simulink model "external_memory_test"  (R2020b)
settings: Solver=FixedStepDiscrete  StartTime=0.0  StopTime=80  RelTol=1e-3
InitFcn:
  | Feature_Width = 64;
  | Feature_Height = 64;
  | Weight_Width = 3;
  | Weight_Height = 3;
  | external_memory_test_init;
values from neighbouring files (symbols this model uses):
  Burst_Length = Feature_Weight_Length    [external_memory_test_init.m]
  byPass = 1    [external_memory_test_init.m]
  Conv_Padding = 0    [external_memory_test_init.m]
  Conv_Stride = 1    [external_memory_test_init.m]
  DDR_Depth = Weight_Length + Feature_Length + outFeature_Length    [external_memory_test_init.m]
  ddrInitData = single((rand(1,DDR_Depth)))    [external_memory_test_init.m]
  Duty_Cycle = 0.5    [external_memory_test_init.m]
  Feature_Area = Feature_Width * Feature_Height    [external_memory_test_init.m]
  Feature_Length = Phase_In * Feature_Area    [external_memory_test_init.m]
  inChannel = 3    [external_memory_test_init.m]
  outChannel = 2    [external_memory_test_init.m]
  outFeature_Length = outFeature_Width * outFeature_Height * Phase_Out    [external_memory_test_init.m]
  Pool_Stride = 2    [external_memory_test_init.m]
  Pool_Width = 2    [external_memory_test_init.m]
  Tc = 1    [external_memory_test_init.m]
  Ti = 1    [external_memory_test_init.m]
  To = 1    [external_memory_test_init.m]
  Tr = 1    [external_memory_test_init.m]
  Weight_Length = Phase_In * Weight_Area * Phase_Out    [external_memory_test_init.m]
undefined symbols (not defined in the file or in its folder): Conv_Step, Pool_Step, sigbuilder_block
libraries: hdlsllib x85, simulink x44, visionhdlutilities x16
(part 1 of 6)
settings Model: DataTypeOverride=Off  Creator=Xiao  LastModifiedBy=Xiao
settings SolverCC: AutoInsertRateTranBlk=on
settings OptimizationCC: BlockReduction=off  ConditionallyExecuteInputs=off  DefaultParameterBehavior=Inlined
settings DebuggingCC: AlgebraicLoopMsg=error  SingleTaskRateTransMsg=error
settings HardwareCC: ProdBitPerPointer=32  ProdBitPerSizeT=32  ProdBitPerPtrDiffT=32  ProdLargestAtomicFloat=None  ProdIntDivRoundTo=Undefined  ProdEndianess=Unspecified  ProdWordSize=32  ProdHWDeviceType=ASIC/FPGA->ASIC/FPGA  TargetBitPerPointer=64  TargetBitPerSizeT=64  TargetBitPerPtrDiffT=64  TargetLongLongMode=on  TargetIntDivRoundTo=Zero  TargetEndianess=LittleEndian  TargetWordSize=64  TargetHWDeviceType=Custom Processor->MATLAB Host Computer  ProdEqTarget=off

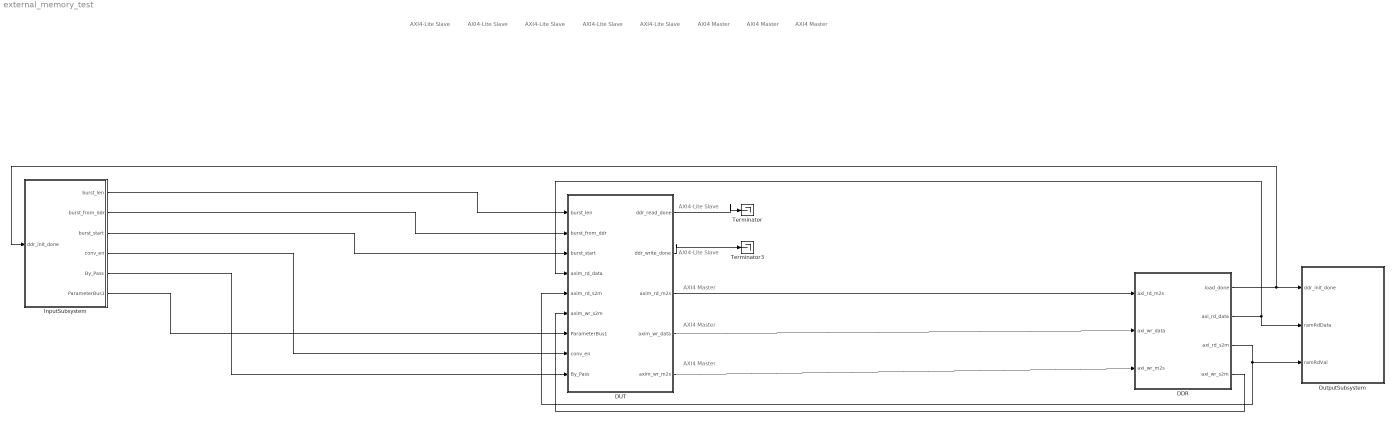
== system external_memory_test ==
  note: AXI4 Master
  note: AXI4-Lite Slave
  note: AXI4-Lite Slave
  note: AXI4-Lite Slave
  note: AXI4 Master
  note: AXI4 Master
  note: AXI4-Lite Slave
  note: AXI4-Lite Slave
  note: AXI4 Master
  note: AXI4-Lite Slave
  note: AXI4 Master
  note: AXI4 Master
  note: AXI4-Lite Slave
  DDR : Subsystem  mask{DDR3_DEPTH=DDR_Depth, INIT_DDR3=on, INIT_ADDR=0, INIT_DATA=ddrInitData(1:DDR_Depth), OutDataTypeStr=uint32, READY_DUTY_CYL=Duty_Cycle, toggle=off}
      mask prompts: DDR3_DEPTH "DDR3 DEPTH"; INIT_DDR3 "Initialize DDR3"; INIT_ADDR "DDR3 Initial Address"; INIT_DATA "DDR3 Initialization data"; OutDataTypeStr "Simulink:blkprm_prompts:UNIFIEDDATATYPE"; READY_DUTY_CYL "READY Duty Cycle"; toggle "Read Valid Toggling"
      mask help: DDR3 Simulation model
      mask init:
      | if(DDR3_DEPTH<=1)
      |     error('DDR size should be greater than 1' )  
      | end
      | 
      | if(READY_DUTY_CYL>1)
      |   error('should be less than 1' )  
      | end
      |    
      | 
      | %%Initialization Value
      | if(INIT_DDR3==true)
      |     if(isempty(INIT_ADDR))
      |      error('Enter Initial address' )  
      |     end   
      | end
      mask Callback INIT_DDR3:
      | % Get the mask parameter values. This is a cell
      | %   array of character vectors.
      | maskStr = get_param(gcb,'INIT_DDR3');
      | 
      | % The pop-up menu is the first mask parameter.
      | %   Check the value selected in the pop-up
      | if strcmp(maskStr,'on')
      | 
      |     % Set the visibility of both parameters on when
      |     %   User-defined is selected in the pop-up.
      | 
      |     set_param(gcb,'MaskEnables',{'on','on','on','on','on','on','on'});
      | 
      | else
      | 
      |     % Turn off the visibility of the Value field
      |     %   when User-defined is not selected.
      | 
      |     set_param(gcb,'MaskEnables',{'on','on','off','off','on','on','on'});
      | 
      |     % Set the character vector in the Values field equal to the
      |     % character vector selected in the Gain pop-up menu.
      | 
      |     %maskStr{2}=maskStr{1};
      | 
      | end
      mask TypeOptions OutDataTypeStr: axi_wr_data/OutDataTypeStr | axi_rd_data/OutDataTypeStr
      mask DialogControl DescGroupVar Prompt: DDR
      mask DialogControl DDR3_INIT Prompt: DDR3 Initialization
      mask DialogControl PARAM_GROUP Prompt: DDR3 Initialization Parameters
      mask DialogControl OutDataTypeStr Prompt: Data type:
      mask DialogControl READY_DUTY_CYL Tooltip: between 0 to 1
  DUT : Subsystem  TreatAsAtomicUnit=on
  InputSubsystem : Subsystem
  OutputSubsystem : Subsystem
  Terminator : Terminator
  Terminator3 : Terminator
  wires:
  DDR/2(axi_rd_data) -> OutputSubsystem/2(ramRdData), DUT/4(axim_rd_data)
  DDR/4(axi_wr_s2m) -> DUT/6(axim_wr_s2m)
  DUT/4(axim_wr_data) -> DDR/2(axi_wr_data)
  DUT/5(axim_wr_m2s) -> DDR/3(axi_wr_m2s)
  DDR/3(axi_rd_s2m) -> OutputSubsystem/3(ramRdVal), DUT/5(axim_rd_s2m)
  DUT/1(ddr_read_done) -> Terminator/1
  DUT/2(ddr_write_done) -> Terminator3/1
  DUT/3(axim_rd_m2s) -> DDR/1(axi_rd_m2s)
  InputSubsystem/2(burst_from_ddr) -> DUT/2(burst_from_ddr)
  InputSubsystem/3(burst_start) -> DUT/3(burst_start)
  InputSubsystem/1(burst_len) -> DUT/1(burst_len)
  DDR/1(load_done) -> OutputSubsystem/1(ddr_init_done), InputSubsystem/1(ddr_init_done)
  InputSubsystem/4(conv_en) -> DUT/8(conv_en)
  InputSubsystem/5(By_Pass) -> DUT/9(By_Pass)
  InputSubsystem/6(ParameterBus1) -> DUT/7(ParameterBus1)

== system external_memory_test/DDR ==
  axi_rd_m2s : Inport
  axi_wr_data : Inport  Port=2  OutDataTypeStr=uint32
  axi_wr_m2s : Inport  Port=3
  Bit Slice1 : hdlsllib/Logic and Bit Operations/Bit Slice  lidx=15  ridx=0
  Bus Creator : BusCreator  Inputs=2
  Bus Creator1 : BusCreator  Inputs=2
  Bus Selector : BusSelector  OutputSignals=rd_addr,rd_len,rd_avalid
  Bus Selector1 : BusSelector  OutputSignals=wr_addr,wr_len,wr_valid
  Constant : Constant  OutDataTypeStr=boolean  SampleTime=-1
  Delay : Delay
  Delay1 : Delay  DelayLength=1
  Delay2 : Delay  DelayLength=1
  Delay3 : Delay  DelayLength=1
  MATLAB System : MATLABSystem  System=hdl.RAM  RAMType=Simple dual port  WriteOutputValue=New data  RAMInitialValue=0  SimulateUsing=Code generation
      mask Type: hdl.RAM
      mask Display:
      | disp(['Simple' char(10) 'Dual Port' char(10) 'RAM']);
      | port_label('input',1,'din');
      | port_label('input',2,'wr_addr');
      | port_label('input',3,'wr_en');
      | port_label('input',4,'rd_addr');
      | port_label('output',1,'rd_dout');
  ddr_ready : Subsystem
  load_init_data : MATLAB Function  TreatAsAtomicUnit=on
  rdLogic : Subsystem
  wrLogic : Subsystem
  wr_addr-3 : Delay  DelayLength=1
  load_done : Outport  VectorParamsAs1DForOutWhenUnconnected=off
  axi_rd_data : Outport  Port=2  OutDataTypeStr=uint32  VectorParamsAs1DForOutWhenUnconnected=off
  axi_rd_s2m : Outport  Port=3  VectorParamsAs1DForOutWhenUnconnected=off
  axi_wr_s2m : Outport  Port=4  VectorParamsAs1DForOutWhenUnconnected=off
  wires:
  Bit Slice1/1 -> wr_addr-3/1
  Delay1/1 -> axi_rd_data/1
  load_init_data/4(ram_wr_enb) -> MATLAB System/3  "ddr_wr_en"
  load_init_data/3(ram_wr_add) -> Bit Slice1/1
  load_init_data/1(load_done) -> ddr_ready/Enable, load_done/1
  MATLAB System/1 -> Delay1/1  "ddr_dout"
  rdLogic/1(ram_rd_addr) -> MATLAB System/4  "ddr_rd_addr"
  wrLogic/1(ram_wr_addr) -> load_init_data/2(axi_wr_add)
  wrLogic/2(ram_wr_enb) -> load_init_data/3(axi_wr_val)
  wr_addr-3/1 -> MATLAB System/2  "ddr_wr_addr"
  Bus Selector/2 -> rdLogic/2(axim_rd_len)  "<rd_len>"
  Bus Selector/1 -> rdLogic/1(axim_rd_addr)  "<rd_addr>"
  Constant/1 -> rdLogic/4(axi_rd_dready)  "<rd_dready>"
  axi_rd_m2s/1 -> Bus Selector/1
  Bus Selector/3 -> rdLogic/3(axim_rd_avalid)  "<rd_avalid>"
  Bus Selector1/1 -> wrLogic/2(axi_addr)  "<wr_addr>"
  axi_wr_m2s/1 -> Delay3/1
  Bus Selector1/3 -> wrLogic/4(axi_wr_enb)  "<wr_valid>"
  Bus Selector1/2 -> wrLogic/3(axi_wr_len)  "<wr_len>"
  rdLogic/2(axim_rd_aready) -> Bus Creator/1  "rd_aready"
  Bus Creator/1 -> axi_rd_s2m/1
  rdLogic/3(axim_rd_dvalid) -> Bus Creator/2  "rd_dvalid"
  ddr_ready/1(rdy_out) -> Delay/1, wrLogic/1(ddr_rdy)
  Bus Creator1/1 -> axi_wr_s2m/1
  wrLogic/3(axi_wr_ack) -> Bus Creator1/2  "wr_complete"
  Delay/1 -> Bus Creator1/1  "wr_ready"
  load_init_data/2(ram_wr_data) -> MATLAB System/1  "ddr_din"
  axi_wr_data/1 -> Delay2/1
  Delay2/1 -> load_init_data/1(axi_wr_data)
  Delay3/1 -> Bus Selector1/1

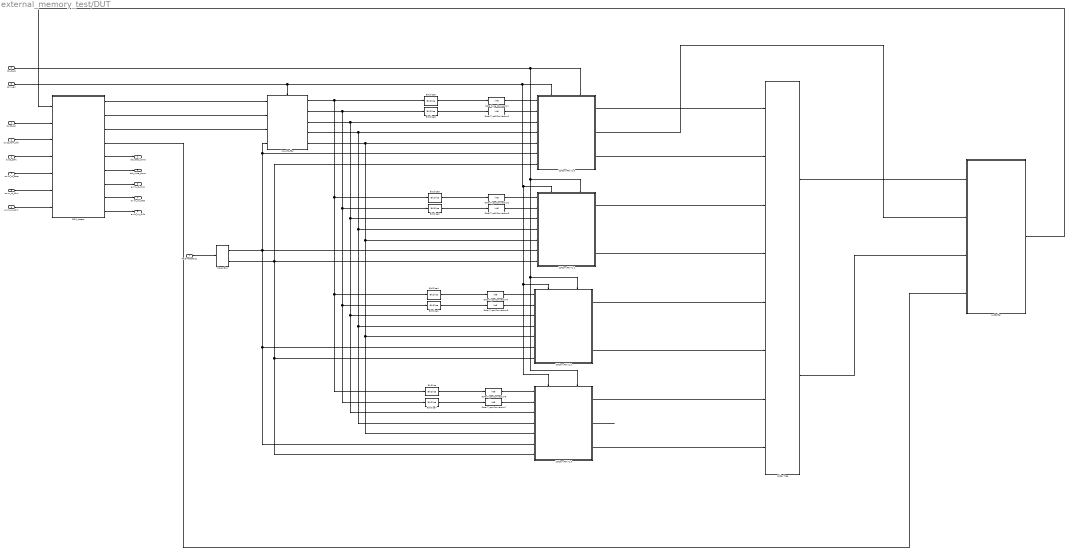
== system external_memory_test/DUT ==
  burst_len : Inport
  burst_from_ddr : Inport  Port=2
  burst_start : Inport  Port=3
  axim_rd_data : Inport  Port=4
  axim_rd_s2m : Inport  Port=5
  axim_wr_s2m : Inport  Port=6
  ParameterBus1 : Inport  Port=7
  conv_en : Inport  Port=8
  By_Pass : Inport  Port=9
  2DConvPE V1.0 : Subsystem
      settings: PortSchema="{\"entries\":[{\"content\":{\"sides\":[{\"content\":{\"connectorIds\":[\"In1\",\"In2\",\"In3\",\"In4\",\"In5\",\"In6\",\"In7\"]},\"type\":\"ConnectorPlacement.EquallySpacedRectSide\",\"uuid\":\"72a132f7-3e47-4ef1-8d79-baadbeb84817\"},{\"content\":{\"connectorIds\":[\"Out1\",\"Out2\",\"Out3\"],\"side\":\"RIGHT\"},\"type\":\"ConnectorPlacement.EquallySpacedRectSide\",\"uuid\":\"2df9bf31-2175-4d97-aafa-a0227f37f2af\"},{\"content\":{\"connectorIds\":[\"In8\",\"In9\"],\"side\":\"TOP\"},\"type\":\"ConnectorPlacement.EquallySpacedRectSide\",\"uuid\":\"1b8495b8-ab7c-42d9-b044-413e20debbac\"},{\"content\":{\"connectorIds\":[],\"side\":\"BOTTOM\"},\"type\":\"ConnectorPlacement.EquallySpacedRectSide\",\"uuid\":\"e68361ac-7f7b-4816-948a-9cecfdd8f729\"},{\"content\":{\"connectorIds\":[],\"side\":\"HIDDEN\"},\"type\":\"ConnectorPlacement.EquallySpacedRectSide\",\"uuid\":\"818be012-dd2c-438f-8537-4d3d95a16bb4\"}]},\"type\":\"ConnectorPlacement.EquallySpacedConnector\",\"uuid\":\"cbadf64c-68f0-4765-b1bf-d60756169ff2\"}],\"packageUris\":[\"http://schema.mathworks.com/mf0/Connector/R2020b\"],\"version\":\"1.0\"}"
  2DConvPE V1.1 : Subsystem
      settings: PortSchema="{\"entries\":[{\"content\":{\"sides\":[{\"content\":{\"connectorIds\":[\"In1\",\"In2\",\"In3\",\"In4\",\"In5\",\"In6\",\"In7\"]},\"type\":\"ConnectorPlacement.EquallySpacedRectSide\",\"uuid\":\"72a132f7-3e47-4ef1-8d79-baadbeb84817\"},{\"content\":{\"connectorIds\":[\"Out1\",\"Out2\",\"Out3\"],\"side\":\"RIGHT\"},\"type\":\"ConnectorPlacement.EquallySpacedRectSide\",\"uuid\":\"2df9bf31-2175-4d97-aafa-a0227f37f2af\"},{\"content\":{\"connectorIds\":[\"In8\",\"In9\"],\"side\":\"TOP\"},\"type\":\"ConnectorPlacement.EquallySpacedRectSide\",\"uuid\":\"1b8495b8-ab7c-42d9-b044-413e20debbac\"},{\"content\":{\"connectorIds\":[],\"side\":\"BOTTOM\"},\"type\":\"ConnectorPlacement.EquallySpacedRectSide\",\"uuid\":\"e68361ac-7f7b-4816-948a-9cecfdd8f729\"},{\"content\":{\"connectorIds\":[],\"side\":\"HIDDEN\"},\"type\":\"ConnectorPlacement.EquallySpacedRectSide\",\"uuid\":\"818be012-dd2c-438f-8537-4d3d95a16bb4\"}]},\"type\":\"ConnectorPlacement.EquallySpacedConnector\",\"uuid\":\"cbadf64c-68f0-4765-b1bf-d60756169ff2\"}],\"packageUris\":[\"http://schema.mathworks.com/mf0/Connector/R2020b\"],\"version\":\"1.0\"}"
  2DConvPE V1.2 : Subsystem
      settings: PortSchema="{\"entries\":[{\"content\":{\"sides\":[{\"content\":{\"connectorIds\":[\"In1\",\"In2\",\"In3\",\"In4\",\"In5\",\"In6\",\"In7\"]},\"type\":\"ConnectorPlacement.EquallySpacedRectSide\",\"uuid\":\"72a132f7-3e47-4ef1-8d79-baadbeb84817\"},{\"content\":{\"connectorIds\":[\"Out1\",\"Out2\",\"Out3\"],\"side\":\"RIGHT\"},\"type\":\"ConnectorPlacement.EquallySpacedRectSide\",\"uuid\":\"2df9bf31-2175-4d97-aafa-a0227f37f2af\"},{\"content\":{\"connectorIds\":[\"In8\",\"In9\"],\"side\":\"TOP\"},\"type\":\"ConnectorPlacement.EquallySpacedRectSide\",\"uuid\":\"1b8495b8-ab7c-42d9-b044-413e20debbac\"},{\"content\":{\"connectorIds\":[],\"side\":\"BOTTOM\"},\"type\":\"ConnectorPlacement.EquallySpacedRectSide\",\"uuid\":\"e68361ac-7f7b-4816-948a-9cecfdd8f729\"},{\"content\":{\"connectorIds\":[],\"side\":\"HIDDEN\"},\"type\":\"ConnectorPlacement.EquallySpacedRectSide\",\"uuid\":\"818be012-dd2c-438f-8537-4d3d95a16bb4\"}]},\"type\":\"ConnectorPlacement.EquallySpacedConnector\",\"uuid\":\"cbadf64c-68f0-4765-b1bf-d60756169ff2\"}],\"packageUris\":[\"http://schema.mathworks.com/mf0/Connector/R2020b\"],\"version\":\"1.0\"}"
  2DConvPE V1.3 : Subsystem
      settings: PortSchema="{\"entries\":[{\"content\":{\"sides\":[{\"content\":{\"connectorIds\":[\"In1\",\"In2\",\"In3\",\"In4\",\"In5\",\"In6\",\"In7\"]},\"type\":\"ConnectorPlacement.EquallySpacedRectSide\",\"uuid\":\"72a132f7-3e47-4ef1-8d79-baadbeb84817\"},{\"content\":{\"connectorIds\":[\"Out1\",\"Out2\",\"Out3\"],\"side\":\"RIGHT\"},\"type\":\"ConnectorPlacement.EquallySpacedRectSide\",\"uuid\":\"2df9bf31-2175-4d97-aafa-a0227f37f2af\"},{\"content\":{\"connectorIds\":[\"In8\",\"In9\"],\"side\":\"TOP\"},\"type\":\"ConnectorPlacement.EquallySpacedRectSide\",\"uuid\":\"1b8495b8-ab7c-42d9-b044-413e20debbac\"},{\"content\":{\"connectorIds\":[],\"side\":\"BOTTOM\"},\"type\":\"ConnectorPlacement.EquallySpacedRectSide\",\"uuid\":\"e68361ac-7f7b-4816-948a-9cecfdd8f729\"},{\"content\":{\"connectorIds\":[],\"side\":\"HIDDEN\"},\"type\":\"ConnectorPlacement.EquallySpacedRectSide\",\"uuid\":\"818be012-dd2c-438f-8537-4d3d95a16bb4\"}]},\"type\":\"ConnectorPlacement.EquallySpacedConnector\",\"uuid\":\"cbadf64c-68f0-4765-b1bf-d60756169ff2\"}],\"packageUris\":[\"http://schema.mathworks.com/mf0/Connector/R2020b\"],\"version\":\"1.0\"}"
  Adder Tree : Subsystem
  Bit Slice : hdlsllib/Logic and Bit Operations/Bit Slice  lidx=7  ridx=0
      settings: SourceProductBaseCode=SL
  Bit Slice1 : hdlsllib/Logic and Bit Operations/Bit Slice  lidx=15  ridx=8
      settings: SourceProductBaseCode=SL
  Bit Slice2 : hdlsllib/Logic and Bit Operations/Bit Slice  lidx=23  ridx=16
      settings: SourceProductBaseCode=SL
  Bit Slice3 : hdlsllib/Logic and Bit Operations/Bit Slice  lidx=31  ridx=24
      settings: SourceProductBaseCode=SL
  Bit Slice4 : hdlsllib/Logic and Bit Operations/Bit Slice  lidx=15  ridx=8
      settings: SourceProductBaseCode=SL
  Bit Slice5 : hdlsllib/Logic and Bit Operations/Bit Slice  lidx=31  ridx=24
      settings: SourceProductBaseCode=SL
  Bit Slice6 : hdlsllib/Logic and Bit Operations/Bit Slice  lidx=31  ridx=24
      settings: SourceProductBaseCode=SL
  Bit Slice7 : hdlsllib/Logic and Bit Operations/Bit Slice  lidx=7  ridx=0
      settings: SourceProductBaseCode=SL
  DDR_Access : Subsystem
  Data Type Conversion{,1..7} (8 alike) : DataTypeConversion  OutDataTypeStr=int8
  Input Buffer : Subsystem
      settings: PortSchema="{\"entries\":[{\"content\":{\"sides\":[{\"content\":{\"connectorIds\":[\"In1\",\"In2\",\"In3\",\"In4\"]},\"type\":\"ConnectorPlacement.EquallySpacedRectSide\",\"uuid\":\"c195afef-7b81-4031-b156-0c076d364d34\"},{\"content\":{\"connectorIds\":[\"Out1\",\"Out2\",\"Out3\",\"Out4\",\"Out5\"],\"side\":\"RIGHT\"},\"type\":\"ConnectorPlacement.EquallySpacedRectSide\",\"uuid\":\"6c59ef52-9ca6-4375-94a4-c9eb63a98ed6\"},{\"content\":{\"connectorIds\":[\"In5\"],\"side\":\"TOP\"},\"type\":\"ConnectorPlacement.EquallySpacedRectSide\",\"uuid\":\"0411db83-8b14-4839-9ba9-9d4adad981fa\"},{\"content\":{\"connectorIds\":[],\"side\":\"BOTTOM\"},\"type\":\"ConnectorPlacement.EquallySpacedRectSide\",\"uuid\":\"b7d3080d-038a-49c2-8bed-119a5f620f56\"},{\"content\":{\"connectorIds\":[],\"side\":\"HIDDEN\"},\"type\":\"ConnectorPlacement.EquallySpacedRectSide\",\"uuid\":\"35581eff-147e-46df-b898-8a30a1508356\"}]},\"type\":\"ConnectorPlacement.EquallySpacedConnector\",\"uuid\":\"e4bcb087-e87d-44d2-a482-8679821b69a7\"}],\"packageUris\":[\"http://schema.mathworks.com/mf0/Connector/R2020b\"],\"version\":\"1.0\"}"
  ParamBus : Subsystem
  outBuffer : Subsystem
  ddr_read_done : Outport  VectorParamsAs1DForOutWhenUnconnected=off
  ddr_write_done : Outport  Port=2  VectorParamsAs1DForOutWhenUnconnected=off
  axim_rd_m2s : Outport  Port=3  VectorParamsAs1DForOutWhenUnconnected=off
  axim_wr_data : Outport  Port=4  VectorParamsAs1DForOutWhenUnconnected=off
  axim_wr_m2s : Outport  Port=5  VectorParamsAs1DForOutWhenUnconnected=off
  wires:
  burst_start/1 -> DDR_Access/4(burst_start)
  DDR_Access/6(ddr_write_done) -> ddr_write_done/1  "ddr_write_done"
  axim_rd_data/1 -> DDR_Access/5(axim_rd_data)
  burst_len/1 -> DDR_Access/2(burst_len)
  burst_from_ddr/1 -> DDR_Access/3(burst_from_ddr)
  DDR_Access/5(ddr_read_done) -> ddr_read_done/1  "ddr_read_done"
  DDR_Access/3(ram_wren) -> Input Buffer/3(ram_wr_en)  "ram_wr_en"
  DDR_Access/1(ram_wr_data) -> Input Buffer/1(ram_wr_data)  "ram_wr_data"
  DDR_Access/7(axim_rd_m2s) -> axim_rd_m2s/1
  DDR_Access/8(axim_wr_data) -> axim_wr_data/1  "axim_wr_data"
  axim_rd_s2m/1 -> DDR_Access/6(axim_rd_s2m)
  axim_wr_s2m/1 -> DDR_Access/7(axim_wr_s2m)
  DDR_Access/9(axim_wr_m2s) -> axim_wr_m2s/1
  DDR_Access/2(ram_wr_addr) -> Input Buffer/2(ram_wr_addr)  "ram_wr_addr"
  conv_en/1 -> 2DConvPE V1.3/8(Conv_en), 2DConvPE V1.2/8(Conv_en), 2DConvPE V1.1/8(Conv_en), 2DConvPE V1.0/8(Conv_en), Input Buffer/5(BufferOut_en)
  Input Buffer/2(feature_data) -> Bit Slice6/1, Bit Slice7/1, Bit Slice1/1, Bit Slice2/1
  Input Buffer/3(feature_data_valid) -> 2DConvPE V1.3/3(Stream_Valid), 2DConvPE V1.2/3(Stream_Valid), 2DConvPE V1.1/3(Stream_Valid), 2DConvPE V1.0/3(Stream_Valid)
  DDR_Access/4(ram_rd_addr) -> outBuffer/4(ram_rd_addr)  "ram_rd_addr"
  outBuffer/1(ram_read_data) -> DDR_Access/1(ram_read_data)
  Input Buffer/4(weight_data_valid) -> 2DConvPE V1.3/4(weight_data_valid), 2DConvPE V1.2/4(weight_data_valid), 2DConvPE V1.1/4(weight_data_valid), 2DConvPE V1.0/4(weight_data_valid)
  Input Buffer/5(PhaseOut_Count) -> 2DConvPE V1.3/5(PhaseOut_Count), 2DConvPE V1.2/5(PhaseOut_Count), 2DConvPE V1.1/5(PhaseOut_Count), 2DConvPE V1.0/5(PhaseOut_Count)
  ParamBus/1(PBus_Conv) -> 2DConvPE V1.3/6(paramBus_Conv), 2DConvPE V1.2/6(paramBus_Conv), 2DConvPE V1.1/6(paramBus_Conv), 2DConvPE V1.0/6(paramBus_Conv), Input Buffer/4(ParamBus_Conv)
  ParamBus/2(PBus_Pool) -> 2DConvPE V1.3/7(paraBus_Pool), 2DConvPE V1.2/7(paraBus_Pool), 2DConvPE V1.1/7(paraBus_Pool), 2DConvPE V1.0/7(paraBus_Pool)
  By_Pass/1 -> 2DConvPE V1.3/9(ByPass), 2DConvPE V1.2/9(ByPass), 2DConvPE V1.1/9(ByPass), 2DConvPE V1.0/9(ByPass)
  2DConvPE V1.0/2(OutAdddess) -> outBuffer/2(ram_wr_addr)
  2DConvPE V1.0/3(OutValid) -> Adder Tree/2(valid1)
  ParameterBus1/1 -> ParamBus/1(ParameterBus1)
  Bit Slice3/1 -> Data Type Conversion2/1
  Bit Slice2/1 -> Data Type Conversion3/1
  Bit Slice6/1 -> Data Type Conversion1/1
  Bit Slice/1 -> Data Type Conversion6/1
  Input Buffer/1(weight_data) -> Bit Slice/1, Bit Slice4/1, Bit Slice3/1, Bit Slice5/1
  Bit Slice5/1 -> Data Type Conversion/1
  Data Type Conversion/1 -> 2DConvPE V1.0/1(weight_data)
  Data Type Conversion1/1 -> 2DConvPE V1.0/2(feature_data)
  Bit Slice7/1 -> Data Type Conversion7/1
  Bit Slice4/1 -> Data Type Conversion4/1
  Bit Slice1/1 -> Data Type Conversion5/1
  2DConvPE V1.1/3(OutValid) -> Adder Tree/4(valid2)
  Data Type Conversion2/1 -> 2DConvPE V1.1/1(weight_data)
  Data Type Conversion3/1 -> 2DConvPE V1.1/2(feature_data)
  Data Type Conversion4/1 -> 2DConvPE V1.2/1(weight_data)
  Data Type Conversion5/1 -> 2DConvPE V1.2/2(feature_data)
  Data Type Conversion6/1 -> 2DConvPE V1.3/1(weight_data)
  Data Type Conversion7/1 -> 2DConvPE V1.3/2(feature_data)
  2DConvPE V1.3/2(OutAdddess) -> ?
  2DConvPE V1.3/3(OutValid) -> Adder Tree/8(valid4)
  2DConvPE V1.2/3(OutValid) -> Adder Tree/6(valid3)
  2DConvPE V1.0/1(OutData) -> Adder Tree/1(In1)
  2DConvPE V1.1/1(OutData) -> Adder Tree/3(In2)
  2DConvPE V1.2/1(OutData) -> Adder Tree/5(In3)
  2DConvPE V1.3/1(OutData) -> Adder Tree/7(In4)
  Adder Tree/1(Out1) -> outBuffer/1(ram_wr_data)
  Adder Tree/2(outvalid) -> outBuffer/3(ram_wr_en)

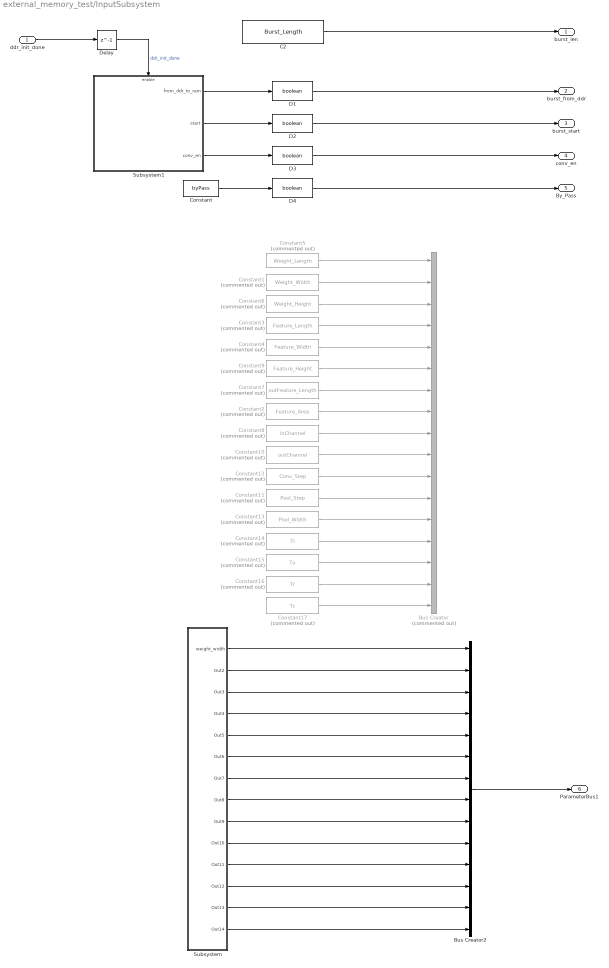
== system external_memory_test/InputSubsystem ==
  ddr_init_done : Inport
  Bus Creator : BusCreator  Commented=on  Inputs=17
  Bus Creator2 : BusCreator  Inputs=14
  C2 : Constant  Value=Burst_Length  OutDataTypeStr=fixdt(0,32,0)  SampleTime=-1
  Constant : Constant  Value=byPass
  Constant1 : Constant  Commented=on  Value=Weight_Width  OutDataTypeStr=uint32  SampleTime=-1
  Constant10 : Constant  Commented=on  Value=outChannel  OutDataTypeStr=uint32  SampleTime=-1
  Constant11 : Constant  Commented=on  Value=Pool_Step  OutDataTypeStr=uint32  SampleTime=-1
  Constant12 : Constant  Commented=on  Value=Conv_Step  OutDataTypeStr=uint32  SampleTime=-1
  Constant13 : Constant  Commented=on  Value=Pool_Width  OutDataTypeStr=uint32  SampleTime=-1
  Constant14 : Constant  Commented=on  Value=Ti  OutDataTypeStr=uint32  SampleTime=-1
  Constant15 : Constant  Commented=on  Value=To  OutDataTypeStr=uint32  SampleTime=-1
  Constant16 : Constant  Commented=on  Value=Tr  OutDataTypeStr=uint32  SampleTime=-1
  Constant17 : Constant  Commented=on  Value=Tc  OutDataTypeStr=uint32  SampleTime=-1
  Constant2 : Constant  Commented=on  Value=Feature_Area  OutDataTypeStr=uint32  SampleTime=-1
  Constant3 : Constant  Commented=on  Value=Feature_Length  OutDataTypeStr=uint32  SampleTime=-1
  Constant4 : Constant  Commented=on  Value=Feature_Width  OutDataTypeStr=uint32  SampleTime=-1
  Constant5 : Constant  Commented=on  Value=Weight_Length  OutDataTypeStr=uint32  SampleTime=-1
  Constant6 : Constant  Commented=on  Value=Weight_Height  OutDataTypeStr=uint32  SampleTime=-1
  Constant7 : Constant  Commented=on  Value=outFeature_Length  OutDataTypeStr=uint32  SampleTime=-1
  Constant8 : Constant  Commented=on  Value=inChannel  OutDataTypeStr=uint32  SampleTime=-1
  Constant9 : Constant  Commented=on  Value=Feature_Height  OutDataTypeStr=uint32  SampleTime=-1
  D{1..4} (4 alike) : DataTypeConversion  OutDataTypeStr=boolean  RndMeth=Simplest
  Delay : Delay  DelayLength=1
  Subsystem : Subsystem
  Subsystem1 : Subsystem
  burst_len : Outport  VectorParamsAs1DForOutWhenUnconnected=off
  burst_from_ddr : Outport  Port=2  VectorParamsAs1DForOutWhenUnconnected=off
  burst_start : Outport  Port=3  VectorParamsAs1DForOutWhenUnconnected=off
  conv_en : Outport  Port=4
  By_Pass : Outport  Port=5
  ParameterBus1 : Outport  Port=6
  wires:
  D1/1 -> burst_from_ddr/1
  C2/1 -> burst_len/1
  Subsystem1/1(from_ddr_to_ram) -> D1/1
  D2/1 -> burst_start/1
  Subsystem1/2(start) -> D2/1
  ddr_init_done/1 -> Delay/1
  Delay/1 -> Subsystem1/Enable  "ddr_init_done"
  Subsystem1/3(conv_en) -> D3/1
  D3/1 -> conv_en/1
  Constant2/1 -> Bus Creator/8
  Constant5/1 -> Bus Creator/1
  Constant1/1 -> Bus Creator/2
  Constant6/1 -> Bus Creator/3
  Constant3/1 -> Bus Creator/4
  Constant4/1 -> Bus Creator/5
  Constant7/1 -> Bus Creator/7
  Constant9/1 -> Bus Creator/6
  Constant8/1 -> Bus Creator/9
  Constant10/1 -> Bus Creator/10
  Constant12/1 -> Bus Creator/11
  Constant11/1 -> Bus Creator/12
  Constant13/1 -> Bus Creator/13
  Constant14/1 -> Bus Creator/14
  Constant15/1 -> Bus Creator/15
  Constant16/1 -> Bus Creator/16
  Constant17/1 -> Bus Creator/17
  Constant/1 -> D4/1
  D4/1 -> By_Pass/1
  Subsystem/2(Out2) -> Bus Creator2/2
  Subsystem/3(Out3) -> Bus Creator2/3
  Subsystem/4(Out4) -> Bus Creator2/4
  Subsystem/5(Out5) -> Bus Creator2/5
  Subsystem/6(Out6) -> Bus Creator2/6
  Subsystem/7(Out7) -> Bus Creator2/7
  Subsystem/8(Out8) -> Bus Creator2/8
  Subsystem/9(Out9) -> Bus Creator2/9
  Subsystem/10(Out10) -> Bus Creator2/10
  Subsystem/11(Out11) -> Bus Creator2/11
  Subsystem/12(Out12) -> Bus Creator2/12
  Subsystem/13(Out13) -> Bus Creator2/13
  Subsystem/14(Out14) -> Bus Creator2/14
  Subsystem/1(weight_width) -> Bus Creator2/1
  Bus Creator2/1 -> ParameterBus1/1

== system external_memory_test/OutputSubsystem ==
  ddr_init_done : Inport
  ramRdData : Inport  Port=2
  ramRdVal : Inport  Port=3
  Bus Selector2 : BusSelector  OutputSignals=rd_dvalid
  to_MATLAB : Subsystem
  wires:
  ddr_init_done/1 -> to_MATLAB/1(ddr_init_done)
  ramRdVal/1 -> Bus Selector2/1
  Bus Selector2/1 -> to_MATLAB/3(ramRdVal)  "<rd_dvalid>"
  ramRdData/1 -> to_MATLAB/2(ramRdData)

== system external_memory_test/DDR/ddr_ready ==
  Enable : EnablePort
  Data Type Conversion : DataTypeConversion  OutDataTypeStr=boolean
  Pulse Generator : DiscretePulseGenerator  Period=1000  PulseWidth=1000 * READY_DUTY_CYL  SampleTime=-1
  rdy_out : Outport  VectorParamsAs1DForOutWhenUnconnected=off
  wires:
  Pulse Generator/1 -> Data Type Conversion/1
  Data Type Conversion/1 -> rdy_out/1

== system external_memory_test/DDR/rdLogic ==
  axim_rd_addr : Inport
  axim_rd_len : Inport  Port=2
  axim_rd_avalid : Inport  Port=3
  axi_rd_dready : Inport  Port=4
  Bit Slice1 : hdlsllib/Logic and Bit Operations/Bit Slice  lidx=15  ridx=0
  Constant : Constant  OutDataTypeStr=boolean  SampleTime=-1
  Delay2 : Delay
  rd_control : MATLAB Function  TreatAsAtomicUnit=on
  ram_rd_addr : Outport  VectorParamsAs1DForOutWhenUnconnected=off
  axim_rd_aready : Outport  Port=2  VectorParamsAs1DForOutWhenUnconnected=off
  axim_rd_dvalid : Outport  Port=3  VectorParamsAs1DForOutWhenUnconnected=off
  wires:
  axim_rd_addr/1 -> rd_control/1(axi_rd_add)
  rd_control/1(ram_rd_addr) -> Bit Slice1/1
  axim_rd_avalid/1 -> rd_control/3(axi_rd_val)
  Bit Slice1/1 -> ram_rd_addr/1
  axi_rd_dready/1 -> rd_control/4(axi_rd_ready)
  Delay2/1 -> axim_rd_dvalid/1
  Constant/1 -> axim_rd_aready/1
  axim_rd_len/1 -> rd_control/2(axi_rd_len)
  rd_control/2(ram_rd_val) -> Delay2/1

== system external_memory_test/DDR/wrLogic ==
  ddr_rdy : Inport
  axi_addr : Inport  Port=2
  axi_wr_len : Inport  Port=3
  axi_wr_enb : Inport  Port=4
  Add : Sum  AccumDataTypeStr=uint32
  Bit Shift : hdlsllib/Logic and Bit Operations/Bit Shift  mode=Shift Right Arithmetic  N=2
      settings: SourceProductName=HDL Coder
  Logical Operator : Logic  Operator=OR  IconShape=distinctive  AllPortsSameDT=off  OutDataTypeStr=boolean
  Wr_control : Subsystem
  ddr_ack_d1 : Delay  DelayLength=1
  ddr_reday_d1 : Delay  DelayLength=1
  ddr_reday_d6 : Delay  DelayLength=4
  ram_wr_addr : Outport  VectorParamsAs1DForOutWhenUnconnected=off
  ram_wr_enb : Outport  Port=2  VectorParamsAs1DForOutWhenUnconnected=off
  axi_wr_ack : Outport  Port=3  VectorParamsAs1DForOutWhenUnconnected=off
  wires:
  Wr_control/1(valAddEnb) -> ram_wr_enb/1
  axi_wr_len/1 -> Wr_control/3(wr_len)
  ddr_rdy/1 -> ddr_reday_d6/1
  axi_addr/1 -> Bit Shift/1
  axi_wr_enb/1 -> Wr_control/2(wr_enb)
  Wr_control/2(axim_ack) -> ddr_ack_d1/1
  Add/1 -> ram_wr_addr/1
  Wr_control/3(ram_addr) -> Add/2
  ddr_reday_d6/1 -> ddr_reday_d1/1, Logical Operator/2
  ddr_ack_d1/1 -> axi_wr_ack/1
  Bit Shift/1 -> Add/1
  ddr_reday_d1/1 -> Logical Operator/1
  Logical Operator/1 -> Wr_control/1(ddr_wr_rdy)

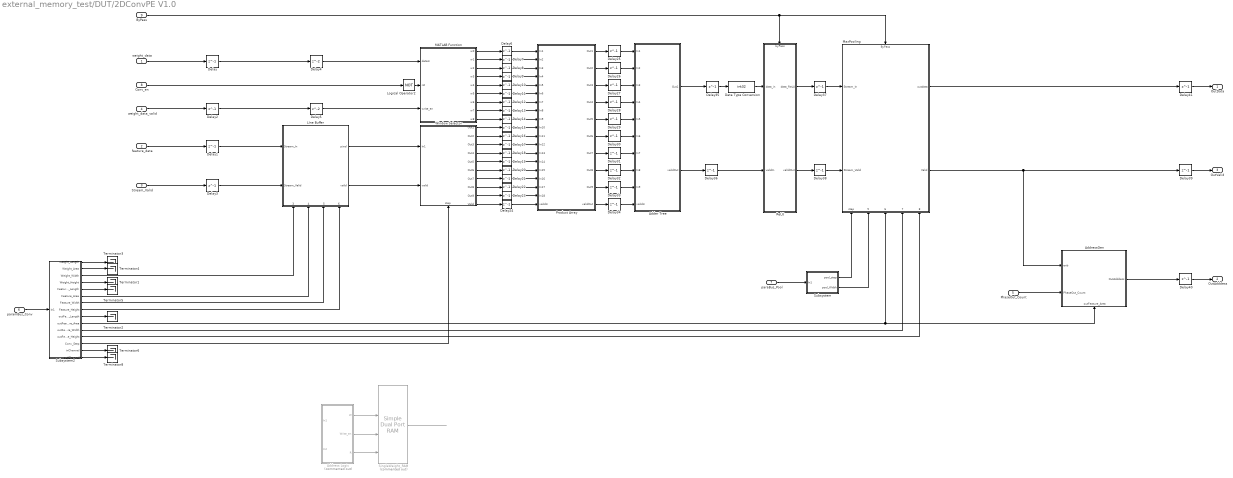
== system external_memory_test/DUT/2DConvPE V1.0 ==
  weight_data : Inport
  feature_data : Inport  Port=2
  Stream_Valid : Inport  Port=3
  weight_data_valid : Inport  Port=4
  PhaseOut_Count : Inport  Port=5
  paramBus_Conv : Inport  Port=6
  paraBus_Pool : Inport  Port=7
  Conv_en : Inport  Port=8
  ByPass : Inport  Port=9
  Adder Tree : Subsystem
  Address Logic : Subsystem  Commented=on
  AddressGen : Subsystem
      settings: PortSchema="{\"entries\":[{\"content\":{\"sides\":[{\"content\":{\"connectorIds\":[\"In1\",\"In2\"]},\"type\":\"ConnectorPlacement.EquallySpacedRectSide\",\"uuid\":\"84e29c71-0390-414b-ab77-a221de5de301\"},{\"content\":{\"connectorIds\":[\"Out1\"],\"side\":\"RIGHT\"},\"type\":\"ConnectorPlacement.EquallySpacedRectSide\",\"uuid\":\"58bcf278-1646-410a-a3e7-26ebbba1e273\"},{\"content\":{\"connectorIds\":[],\"side\":\"TOP\"},\"type\":\"ConnectorPlacement.EquallySpacedRectSide\",\"uuid\":\"d4babae5-c4b0-401f-9df6-cdd80e926352\"},{\"content\":{\"connectorIds\":[\"In3\"],\"side\":\"BOTTOM\"},\"type\":\"ConnectorPlacement.EquallySpacedRectSide\",\"uuid\":\"a08cab3a-dc4c-4404-aa4b-33dfd1f89102\"},{\"content\":{\"connectorIds\":[],\"side\":\"HIDDEN\"},\"type\":\"ConnectorPlacement.EquallySpacedRectSide\",\"uuid\":\"888452d7-95df-443f-995a-66331a7f8c73\"}]},\"type\":\"ConnectorPlacement.EquallySpacedConnector\",\"uuid\":\"691e5dfa-d85a-42aa-a608-f1539775aaa8\"}],\"packageUris\":[\"http://schema.mathworks.com/mf0/Connector/R2020b\"],\"version\":\"1.0\"}"
  Data Type Conversion : DataTypeConversion  OutDataTypeStr=int32
  Delay{,1..3,6..41} (40 alike) : Delay  DelayLength=1
  Delay4 : Delay
  Delay5 : Delay
  LIne Buffer : Subsystem
      settings: PortSchema="{\"entries\":[{\"content\":{\"sides\":[{\"content\":{\"connectorIds\":[\"In1\",\"In2\"]},\"type\":\"ConnectorPlacement.EquallySpacedRectSide\",\"uuid\":\"a250c848-7a40-462c-bfcf-0ff48046d99d\"},{\"content\":{\"connectorIds\":[\"Out1\",\"Out2\"],\"side\":\"RIGHT\"},\"type\":\"ConnectorPlacement.EquallySpacedRectSide\",\"uuid\":\"81aecf2d-6bfb-4d40-80c7-cfb89c921406\"},{\"content\":{\"connectorIds\":[],\"side\":\"TOP\"},\"type\":\"ConnectorPlacement.EquallySpacedRectSide\",\"uuid\":\"288ccc7a-b219-4526-a408-3d8b1082f4b0\"},{\"content\":{\"connectorIds\":[\"In3\",\"In4\",\"In5\",\"In6\"],\"side\":\"BOTTOM\"},\"type\":\"ConnectorPlacement.EquallySpacedRectSide\",\"uuid\":\"5d9529f5-ee70-4412-83ca-b280a2219284\"},{\"content\":{\"connectorIds\":[],\"side\":\"HIDDEN\"},\"type\":\"ConnectorPlacement.EquallySpacedRectSide\",\"uuid\":\"3d06d450-49b0-49ba-a273-690d97c3e8e1\"}]},\"type\":\"ConnectorPlacement.EquallySpacedConnector\",\"uuid\":\"b82e05d1-4695-4e04-9663-17698b30471b\"}],\"packageUris\":[\"http://schema.mathworks.com/mf0/Connector/R2020b\"],\"version\":\"1.0\"}"
  Logical Operator2 : Logic  Operator=NOT  AllPortsSameDT=off  OutDataTypeStr=boolean
  MATLAB Function : MATLAB Function  TreatAsAtomicUnit=on
  MaxPooling : Subsystem
      settings: PortSchema="{\"entries\":[{\"content\":{\"sides\":[{\"content\":{\"connectorIds\":[\"In1\",\"In2\"]},\"type\":\"ConnectorPlacement.EquallySpacedRectSide\",\"uuid\":\"8f082555-10a5-4426-9c6d-30ad9c9edc83\"},{\"content\":{\"connectorIds\":[\"Out1\",\"Out2\"],\"side\":\"RIGHT\"},\"type\":\"ConnectorPlacement.EquallySpacedRectSide\",\"uuid\":\"2f08e48d-98a7-49ef-9240-49e9a92f7835\"},{\"content\":{\"connectorIds\":[\"In3\"],\"side\":\"TOP\"},\"type\":\"ConnectorPlacement.EquallySpacedRectSide\",\"uuid\":\"9c785374-bdb9-47d6-a84c-95016a7dac24\"},{\"content\":{\"connectorIds\":[\"In4\",\"In5\",\"In6\",\"In7\",\"In8\"],\"side\":\"BOTTOM\"},\"type\":\"ConnectorPlacement.EquallySpacedRectSide\",\"uuid\":\"81220b33-16bc-4efc-91f7-9bf9738f949c\"},{\"content\":{\"connectorIds\":[],\"side\":\"HIDDEN\"},\"type\":\"ConnectorPlacement.EquallySpacedRectSide\",\"uuid\":\"99d22b10-fe8c-4c64-8a09-c433657226d7\"}]},\"type\":\"ConnectorPlacement.EquallySpacedConnector\",\"uuid\":\"f09d9050-86eb-4a30-82a2-eebdb84e68d3\"}],\"packageUris\":[\"http://schema.mathworks.com/mf0/Connector/R2020b\"],\"version\":\"1.0\"}"
  Product Array : Subsystem
  ReLU : Subsystem
      settings: PortSchema="{\"entries\":[{\"content\":{\"sides\":[{\"content\":{\"connectorIds\":[\"In1\",\"In2\"]},\"type\":\"ConnectorPlacement.EquallySpacedRectSide\",\"uuid\":\"abc19905-3b44-4985-b45b-942e5eaa1386\"},{\"content\":{\"connectorIds\":[\"Out1\",\"Out2\"],\"side\":\"RIGHT\"},\"type\":\"ConnectorPlacement.EquallySpacedRectSide\",\"uuid\":\"b0a86706-72e5-448b-9f1b-a0967f50aac9\"},{\"content\":{\"connectorIds\":[\"In3\"],\"side\":\"TOP\"},\"type\":\"ConnectorPlacement.EquallySpacedRectSide\",\"uuid\":\"df5d57b0-52e5-439f-8896-63a90ec5378c\"},{\"content\":{\"connectorIds\":[],\"side\":\"HIDDEN\"},\"type\":\"ConnectorPlacement.EquallySpacedRectSide\",\"uuid\":\"493b8843-365c-4ea1-b4d2-a52d72a7a785\"}]},\"type\":\"ConnectorPlacement.EquallySpacedConnector\",\"uuid\":\"755c5668-4a5f-4120-9a22-1155c417e52d\"}],\"packageUris\":[\"http://schema.mathworks.com/mf0/Connector/R2020b\"],\"version\":\"1.0\"}"
  SingleWeight_RAM : hdlsllib/HDL RAMs/Simple Dual Port RAM  Commented=on  ram_size=13
      settings: SourceProductName=HDL Coder
  Subsystem : Subsystem
  Subsystem2 : Subsystem
  Terminator{1..6,8} (7 alike) : Terminator
  Window Selector : Subsystem
      settings: PortSchema="{\"entries\":[{\"content\":{\"sides\":[{\"content\":{\"connectorIds\":[\"In1\",\"In2\"]},\"type\":\"ConnectorPlacement.EquallySpacedRectSide\",\"uuid\":\"2f98ee57-d732-418e-86bd-7acbaf2524e0\"},{\"content\":{\"connectorIds\":[\"Out1\",\"Out2\",\"Out3\",\"Out4\",\"Out5\",\"Out6\",\"Out7\",\"Out8\",\"Out9\",\"Out10\"],\"side\":\"RIGHT\"},\"type\":\"ConnectorPlacement.EquallySpacedRectSide\",\"uuid\":\"287ad403-178f-48f1-9791-2ccad363e9c6\"},{\"content\":{\"connectorIds\":[],\"side\":\"TOP\"},\"type\":\"ConnectorPlacement.EquallySpacedRectSide\",\"uuid\":\"a860ecae-5cde-45ef-a487-fdb4fb7390aa\"},{\"content\":{\"connectorIds\":[\"In3\"],\"side\":\"BOTTOM\"},\"type\":\"ConnectorPlacement.EquallySpacedRectSide\",\"uuid\":\"925435f5-0fb8-4a67-9f76-fe99b5b92634\"},{\"content\":{\"connectorIds\":[],\"side\":\"HIDDEN\"},\"type\":\"ConnectorPlacement.EquallySpacedRectSide\",\"uuid\":\"e6f3edac-a41a-4276-8ae6-cd8be9b02af9\"}]},\"type\":\"ConnectorPlacement.EquallySpacedConnector\",\"uuid\":\"0e32a9d0-da82-46c8-ab50-9de41c4380a9\"}],\"packageUris\":[\"http://schema.mathworks.com/mf0/Connector/R2020b\"],\"version\":\"1.0\"}"
  OutData : Outport
  OutAdddess : Outport  Port=2
  OutValid : Outport  Port=3
  wires:
  Delay/1 -> Delay4/1
  Address Logic/1(W) -> SingleWeight_RAM/2
  Address Logic/2(Write_en) -> SingleWeight_RAM/3
  Address Logic/3(R) -> SingleWeight_RAM/4
  SingleWeight_RAM/1 -> ?
  Conv_en/1 -> Logical Operator2/1
  Delay2/1 -> Delay5/1
  Logical Operator2/1 -> MATLAB Function/2(rst)
  AddressGen/1(OutAdddess) -> Delay40/1
  Adder Tree/1(Out1) -> Delay35/1
  Data Type Conversion/1 -> ReLU/1(data_in)
  ReLU/1(data_ReLU) -> Delay37/1
  PhaseOut_Count/1 -> AddressGen/2(PhaseOut_Count)
  ByPass/1 -> MaxPooling/3(ByPass), ReLU/3(byPass)
  MaxPooling/1(outdata) -> Delay41/1
  MaxPooling/2(Valid) -> Delay39/1, AddressGen/1(enb)
  paraBus_Pool/1 -> Subsystem/1(In1)
  Subsystem/1(pool_step) -> MaxPooling/4(step)
  Subsystem/2(pool_Width) -> MaxPooling/5(Window_Width)
  Subsystem2/11(outFeature_Width) -> MaxPooling/7(Feature_Width)
  Subsystem2/10(outFeature_Area) -> MaxPooling/6(Feature_Area), AddressGen/3(outFeature_Area)
  Subsystem2/12(outFeature_Height) -> MaxPooling/8(Feature_Height)
  paramBus_Conv/1 -> Subsystem2/1(In1)
  Subsystem2/14(inChannel) -> Terminator6/1
  Subsystem2/4(Weight_Height) -> Terminator1/1
  Subsystem2/9(outFeature_Length) -> Terminator2/1
  Subsystem2/13(Conv_Step) -> Window Selector/3(step)
  Subsystem2/1(Weight_Length) -> Terminator3/1
  Subsystem2/2(Weight_Area) -> Terminator4/1
  Subsystem2/5(Feature_Length) -> Terminator5/1
  Subsystem2/15(outChannel) -> Terminator8/1
  Adder Tree/2(validOut) -> Delay36/1
  ReLU/2(valildOut) -> Delay38/1
  Delay1/1 -> LIne Buffer/1(Stream_In)
  Delay3/1 -> LIne Buffer/2(Stream_Valid)
  Subsystem2/3(Weight_Width) -> LIne Buffer/3(Weight_Width)
  Subsystem2/6(Feature_Area) -> LIne Buffer/4(Feature_Area)
  Subsystem2/7(Feature_Width) -> LIne Buffer/5(Feature_Width)
  Subsystem2/8(Feature_Height) -> LIne Buffer/6(Feature_Height)
  LIne Buffer/1(pixel) -> Window Selector/1(In1)
  LIne Buffer/2(valid) -> Window Selector/2(valid)
  weight_data/1 -> Delay/1
  weight_data_valid/1 -> Delay2/1
  feature_data/1 -> Delay1/1
  Stream_Valid/1 -> Delay3/1
  Delay5/1 -> MATLAB Function/3(write_en)
  Delay4/1 -> MATLAB Function/1(dataIn)
  MATLAB Function/1(w0) -> Delay6/1
  Delay6/1 -> Product Array/1(In1)
  MATLAB Function/2(w1) -> Delay7/1
  Delay7/1 -> Product Array/2(In2)
  MATLAB Function/3(w2) -> Delay8/1
  Delay8/1 -> Product Array/3(In3)
  MATLAB Function/4(w3) -> Delay9/1
  Delay9/1 -> Product Array/4(In4)
  MATLAB Function/5(w4) -> Delay10/1
  Delay10/1 -> Product Array/5(In5)
  MATLAB Function/6(w5) -> Delay11/1
  Delay11/1 -> Product Array/6(In6)
  MATLAB Function/7(w6) -> Delay12/1
  Delay12/1 -> Product Array/7(In7)
  MATLAB Function/8(w7) -> Delay13/1
  Delay13/1 -> Product Array/8(In8)
  MATLAB Function/9(w8) -> Delay14/1
  Delay14/1 -> Product Array/9(In9)
  Window Selector/1(Out1) -> Delay15/1
  Delay15/1 -> Product Array/10(In10)
  Window Selector/2(Out2) -> Delay16/1
  Delay16/1 -> Product Array/11(In11)
  Window Selector/3(Out3) -> Delay17/1
  Delay17/1 -> Product Array/12(In12)
  Window Selector/4(Out4) -> Delay18/1
  Delay18/1 -> Product Array/13(In13)
  Window Selector/5(Out5) -> Delay19/1
  Delay19/1 -> Product Array/14(In14)
  Window Selector/6(Out6) -> Delay20/1
  Delay20/1 -> Product Array/15(In15)
  Window Selector/7(Out7) -> Delay21/1
  Delay21/1 -> Product Array/16(In16)
  Window Selector/8(Out8) -> Delay22/1
  Delay22/1 -> Product Array/17(In17)
  Window Selector/9(Out9) -> Delay23/1
  Delay23/1 -> Product Array/18(In18)
  Window Selector/10(Valid) -> Delay24/1
  Delay24/1 -> Product Array/19(validIn)
  Product Array/1(Out1) -> Delay25/1
  Delay25/1 -> Adder Tree/1(In1)
  Product Array/2(Out2) -> Delay26/1
  Product Array/3(Out3) -> Delay27/1
  Product Array/4(Out4) -> Delay28/1
  Product Array/5(Out5) -> Delay29/1
  Product Array/6(Out6) -> Delay30/1
  Product Array/7(Out7) -> Delay31/1
  Product Array/9(Out9) -> Delay33/1
  Product Array/8(Out8) -> Delay32/1
  Product Array/10(validOut) -> Delay34/1
  Delay26/1 -> Adder Tree/2(In2)
  Delay27/1 -> Adder Tree/3(In3)
  Delay28/1 -> Adder Tree/4(In4)
  Delay29/1 -> Adder Tree/5(In5)
  Delay30/1 -> Adder Tree/6(In6)
  Delay31/1 -> Adder Tree/7(In7)
  Delay32/1 -> Adder Tree/8(In8)
  Delay33/1 -> Adder Tree/9(In9)
  Delay34/1 -> Adder Tree/10(validIn)
  Delay35/1 -> Data Type Conversion/1
  Delay36/1 -> ReLU/2(validIn)
  Delay37/1 -> MaxPooling/1(Stream_In)
  Delay38/1 -> MaxPooling/2(Stream_Valid)
  Delay41/1 -> OutData/1
  Delay39/1 -> OutValid/1
  Delay40/1 -> OutAdddess/1

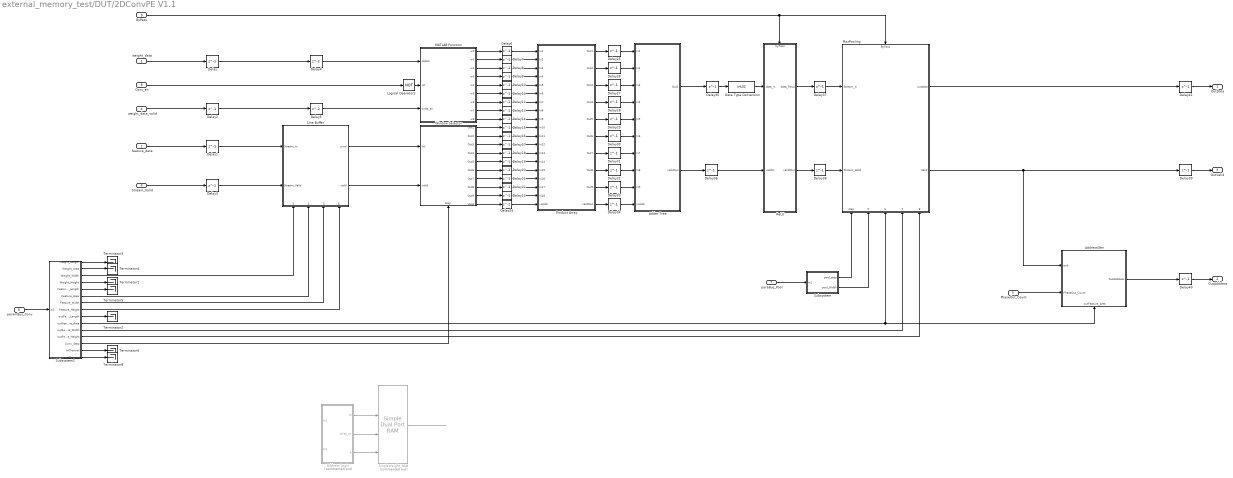
== system external_memory_test/DUT/2DConvPE V1.1 ==
  weight_data : Inport
  feature_data : Inport  Port=2
  Stream_Valid : Inport  Port=3
  weight_data_valid : Inport  Port=4
  PhaseOut_Count : Inport  Port=5
  paramBus_Conv : Inport  Port=6
  paraBus_Pool : Inport  Port=7
  Conv_en : Inport  Port=8
  ByPass : Inport  Port=9
  Adder Tree : Subsystem
  Address Logic : Subsystem  Commented=on
  AddressGen : Subsystem
      settings: PortSchema="{\"entries\":[{\"content\":{\"sides\":[{\"content\":{\"connectorIds\":[\"In1\",\"In2\"]},\"type\":\"ConnectorPlacement.EquallySpacedRectSide\",\"uuid\":\"84e29c71-0390-414b-ab77-a221de5de301\"},{\"content\":{\"connectorIds\":[\"Out1\"],\"side\":\"RIGHT\"},\"type\":\"ConnectorPlacement.EquallySpacedRectSide\",\"uuid\":\"58bcf278-1646-410a-a3e7-26ebbba1e273\"},{\"content\":{\"connectorIds\":[],\"side\":\"TOP\"},\"type\":\"ConnectorPlacement.EquallySpacedRectSide\",\"uuid\":\"d4babae5-c4b0-401f-9df6-cdd80e926352\"},{\"content\":{\"connectorIds\":[\"In3\"],\"side\":\"BOTTOM\"},\"type\":\"ConnectorPlacement.EquallySpacedRectSide\",\"uuid\":\"a08cab3a-dc4c-4404-aa4b-33dfd1f89102\"},{\"content\":{\"connectorIds\":[],\"side\":\"HIDDEN\"},\"type\":\"ConnectorPlacement.EquallySpacedRectSide\",\"uuid\":\"888452d7-95df-443f-995a-66331a7f8c73\"}]},\"type\":\"ConnectorPlacement.EquallySpacedConnector\",\"uuid\":\"691e5dfa-d85a-42aa-a608-f1539775aaa8\"}],\"packageUris\":[\"http://schema.mathworks.com/mf0/Connector/R2020b\"],\"version\":\"1.0\"}"
  Data Type Conversion : DataTypeConversion  OutDataTypeStr=int32
  Delay{,1..3,6..41} (40 alike) : Delay  DelayLength=1
  Delay4 : Delay
  Delay5 : Delay
  LIne Buffer : Subsystem
      settings: PortSchema="{\"entries\":[{\"content\":{\"sides\":[{\"content\":{\"connectorIds\":[\"In1\",\"In2\"]},\"type\":\"ConnectorPlacement.EquallySpacedRectSide\",\"uuid\":\"a250c848-7a40-462c-bfcf-0ff48046d99d\"},{\"content\":{\"connectorIds\":[\"Out1\",\"Out2\"],\"side\":\"RIGHT\"},\"type\":\"ConnectorPlacement.EquallySpacedRectSide\",\"uuid\":\"81aecf2d-6bfb-4d40-80c7-cfb89c921406\"},{\"content\":{\"connectorIds\":[],\"side\":\"TOP\"},\"type\":\"ConnectorPlacement.EquallySpacedRectSide\",\"uuid\":\"288ccc7a-b219-4526-a408-3d8b1082f4b0\"},{\"content\":{\"connectorIds\":[\"In3\",\"In4\",\"In5\",\"In6\"],\"side\":\"BOTTOM\"},\"type\":\"ConnectorPlacement.EquallySpacedRectSide\",\"uuid\":\"5d9529f5-ee70-4412-83ca-b280a2219284\"},{\"content\":{\"connectorIds\":[],\"side\":\"HIDDEN\"},\"type\":\"ConnectorPlacement.EquallySpacedRectSide\",\"uuid\":\"3d06d450-49b0-49ba-a273-690d97c3e8e1\"}]},\"type\":\"ConnectorPlacement.EquallySpacedConnector\",\"uuid\":\"b82e05d1-4695-4e04-9663-17698b30471b\"}],\"packageUris\":[\"http://schema.mathworks.com/mf0/Connector/R2020b\"],\"version\":\"1.0\"}"
  Logical Operator2 : Logic  Operator=NOT  AllPortsSameDT=off  OutDataTypeStr=boolean
  MATLAB Function : MATLAB Function  TreatAsAtomicUnit=on
  MaxPooling : Subsystem
      settings: PortSchema="{\"entries\":[{\"content\":{\"sides\":[{\"content\":{\"connectorIds\":[\"In1\",\"In2\"]},\"type\":\"ConnectorPlacement.EquallySpacedRectSide\",\"uuid\":\"8f082555-10a5-4426-9c6d-30ad9c9edc83\"},{\"content\":{\"connectorIds\":[\"Out1\",\"Out2\"],\"side\":\"RIGHT\"},\"type\":\"ConnectorPlacement.EquallySpacedRectSide\",\"uuid\":\"2f08e48d-98a7-49ef-9240-49e9a92f7835\"},{\"content\":{\"connectorIds\":[\"In3\"],\"side\":\"TOP\"},\"type\":\"ConnectorPlacement.EquallySpacedRectSide\",\"uuid\":\"9c785374-bdb9-47d6-a84c-95016a7dac24\"},{\"content\":{\"connectorIds\":[\"In4\",\"In5\",\"In6\",\"In7\",\"In8\"],\"side\":\"BOTTOM\"},\"type\":\"ConnectorPlacement.EquallySpacedRectSide\",\"uuid\":\"81220b33-16bc-4efc-91f7-9bf9738f949c\"},{\"content\":{\"connectorIds\":[],\"side\":\"HIDDEN\"},\"type\":\"ConnectorPlacement.EquallySpacedRectSide\",\"uuid\":\"99d22b10-fe8c-4c64-8a09-c433657226d7\"}]},\"type\":\"ConnectorPlacement.EquallySpacedConnector\",\"uuid\":\"f09d9050-86eb-4a30-82a2-eebdb84e68d3\"}],\"packageUris\":[\"http://schema.mathworks.com/mf0/Connector/R2020b\"],\"version\":\"1.0\"}"
  Product Array : Subsystem
  ReLU : Subsystem
      settings: PortSchema="{\"entries\":[{\"content\":{\"sides\":[{\"content\":{\"connectorIds\":[\"In1\",\"In2\"]},\"type\":\"ConnectorPlacement.EquallySpacedRectSide\",\"uuid\":\"abc19905-3b44-4985-b45b-942e5eaa1386\"},{\"content\":{\"connectorIds\":[\"Out1\",\"Out2\"],\"side\":\"RIGHT\"},\"type\":\"ConnectorPlacement.EquallySpacedRectSide\",\"uuid\":\"b0a86706-72e5-448b-9f1b-a0967f50aac9\"},{\"content\":{\"connectorIds\":[\"In3\"],\"side\":\"TOP\"},\"type\":\"ConnectorPlacement.EquallySpacedRectSide\",\"uuid\":\"df5d57b0-52e5-439f-8896-63a90ec5378c\"},{\"content\":{\"connectorIds\":[],\"side\":\"HIDDEN\"},\"type\":\"ConnectorPlacement.EquallySpacedRectSide\",\"uuid\":\"493b8843-365c-4ea1-b4d2-a52d72a7a785\"}]},\"type\":\"ConnectorPlacement.EquallySpacedConnector\",\"uuid\":\"755c5668-4a5f-4120-9a22-1155c417e52d\"}],\"packageUris\":[\"http://schema.mathworks.com/mf0/Connector/R2020b\"],\"version\":\"1.0\"}"
  SingleWeight_RAM : hdlsllib/HDL RAMs/Simple Dual Port RAM  Commented=on  ram_size=13
      settings: SourceProductName=HDL Coder
  Subsystem : Subsystem
  Subsystem2 : Subsystem
  Terminator{1..6,8} (7 alike) : Terminator
  Window Selector : Subsystem
      settings: PortSchema="{\"entries\":[{\"content\":{\"sides\":[{\"content\":{\"connectorIds\":[\"In1\",\"In2\"]},\"type\":\"ConnectorPlacement.EquallySpacedRectSide\",\"uuid\":\"2f98ee57-d732-418e-86bd-7acbaf2524e0\"},{\"content\":{\"connectorIds\":[\"Out1\",\"Out2\",\"Out3\",\"Out4\",\"Out5\",\"Out6\",\"Out7\",\"Out8\",\"Out9\",\"Out10\"],\"side\":\"RIGHT\"},\"type\":\"ConnectorPlacement.EquallySpacedRectSide\",\"uuid\":\"287ad403-178f-48f1-9791-2ccad363e9c6\"},{\"content\":{\"connectorIds\":[],\"side\":\"TOP\"},\"type\":\"ConnectorPlacement.EquallySpacedRectSide\",\"uuid\":\"a860ecae-5cde-45ef-a487-fdb4fb7390aa\"},{\"content\":{\"connectorIds\":[\"In3\"],\"side\":\"BOTTOM\"},\"type\":\"ConnectorPlacement.EquallySpacedRectSide\",\"uuid\":\"925435f5-0fb8-4a67-9f76-fe99b5b92634\"},{\"content\":{\"connectorIds\":[],\"side\":\"HIDDEN\"},\"type\":\"ConnectorPlacement.EquallySpacedRectSide\",\"uuid\":\"e6f3edac-a41a-4276-8ae6-cd8be9b02af9\"}]},\"type\":\"ConnectorPlacement.EquallySpacedConnector\",\"uuid\":\"0e32a9d0-da82-46c8-ab50-9de41c4380a9\"}],\"packageUris\":[\"http://schema.mathworks.com/mf0/Connector/R2020b\"],\"version\":\"1.0\"}"
  OutData : Outport
  OutAdddess : Outport  Port=2
  OutValid : Outport  Port=3
  wires:
  Delay/1 -> Delay4/1
  Address Logic/1(W) -> SingleWeight_RAM/2
  Address Logic/2(Write_en) -> SingleWeight_RAM/3
  Address Logic/3(R) -> SingleWeight_RAM/4
  SingleWeight_RAM/1 -> ?
  Conv_en/1 -> Logical Operator2/1
  Delay2/1 -> Delay5/1
  Logical Operator2/1 -> MATLAB Function/2(rst)
  AddressGen/1(OutAdddess) -> Delay40/1
  Adder Tree/1(Out1) -> Delay35/1
  Data Type Conversion/1 -> ReLU/1(data_in)
  ReLU/1(data_ReLU) -> Delay37/1
  PhaseOut_Count/1 -> AddressGen/2(PhaseOut_Count)
  ByPass/1 -> MaxPooling/3(ByPass), ReLU/3(byPass)
  MaxPooling/1(outdata) -> Delay41/1
  MaxPooling/2(Valid) -> Delay39/1, AddressGen/1(enb)
  paraBus_Pool/1 -> Subsystem/1(In1)
  Subsystem/1(pool_step) -> MaxPooling/4(step)
  Subsystem/2(pool_Width) -> MaxPooling/5(Window_Width)
  Subsystem2/11(outFeature_Width) -> MaxPooling/7(Feature_Width)
  Subsystem2/10(outFeature_Area) -> MaxPooling/6(Feature_Area), AddressGen/3(outFeature_Area)
  Subsystem2/12(outFeature_Height) -> MaxPooling/8(Feature_Height)
  paramBus_Conv/1 -> Subsystem2/1(In1)
  Subsystem2/14(inChannel) -> Terminator6/1
  Subsystem2/4(Weight_Height) -> Terminator1/1
  Subsystem2/9(outFeature_Length) -> Terminator2/1
  Subsystem2/13(Conv_Step) -> Window Selector/3(step)
  Subsystem2/1(Weight_Length) -> Terminator3/1
  Subsystem2/2(Weight_Area) -> Terminator4/1
  Subsystem2/5(Feature_Length) -> Terminator5/1
  Subsystem2/15(outChannel) -> Terminator8/1
  Adder Tree/2(validOut) -> Delay36/1
  ReLU/2(valildOut) -> Delay38/1
  Delay1/1 -> LIne Buffer/1(Stream_In)
  Delay3/1 -> LIne Buffer/2(Stream_Valid)
  Subsystem2/3(Weight_Width) -> LIne Buffer/3(Weight_Width)
  Subsystem2/6(Feature_Area) -> LIne Buffer/4(Feature_Area)
  Subsystem2/7(Feature_Width) -> LIne Buffer/5(Feature_Width)
  Subsystem2/8(Feature_Height) -> LIne Buffer/6(Feature_Height)
  LIne Buffer/1(pixel) -> Window Selector/1(In1)
  LIne Buffer/2(valid) -> Window Selector/2(valid)
  weight_data/1 -> Delay/1
  weight_data_valid/1 -> Delay2/1
  feature_data/1 -> Delay1/1
  Stream_Valid/1 -> Delay3/1
  Delay5/1 -> MATLAB Function/3(write_en)
  Delay4/1 -> MATLAB Function/1(dataIn)
  MATLAB Function/1(w0) -> Delay6/1
  Delay6/1 -> Product Array/1(In1)
  MATLAB Function/2(w1) -> Delay7/1
  Delay7/1 -> Product Array/2(In2)
  MATLAB Function/3(w2) -> Delay8/1
  Delay8/1 -> Product Array/3(In3)
  MATLAB Function/4(w3) -> Delay9/1
  Delay9/1 -> Product Array/4(In4)
  MATLAB Function/5(w4) -> Delay10/1
  Delay10/1 -> Product Array/5(In5)
  MATLAB Function/6(w5) -> Delay11/1
  Delay11/1 -> Product Array/6(In6)
  MATLAB Function/7(w6) -> Delay12/1
  Delay12/1 -> Product Array/7(In7)
  MATLAB Function/8(w7) -> Delay13/1
  Delay13/1 -> Product Array/8(In8)
  MATLAB Function/9(w8) -> Delay14/1
  Delay14/1 -> Product Array/9(In9)
  Window Selector/1(Out1) -> Delay15/1
  Delay15/1 -> Product Array/10(In10)
  Window Selector/2(Out2) -> Delay16/1
  Delay16/1 -> Product Array/11(In11)
  Window Selector/3(Out3) -> Delay17/1
  Delay17/1 -> Product Array/12(In12)
  Window Selector/4(Out4) -> Delay18/1
  Delay18/1 -> Product Array/13(In13)
  Window Selector/5(Out5) -> Delay19/1
  Delay19/1 -> Product Array/14(In14)
  Window Selector/6(Out6) -> Delay20/1
  Delay20/1 -> Product Array/15(In15)
  Window Selector/7(Out7) -> Delay21/1
  Delay21/1 -> Product Array/16(In16)
  Window Selector/8(Out8) -> Delay22/1
  Delay22/1 -> Product Array/17(In17)
  Window Selector/9(Out9) -> Delay23/1
  Delay23/1 -> Product Array/18(In18)
  Window Selector/10(Valid) -> Delay24/1
  Delay24/1 -> Product Array/19(validIn)
  Product Array/1(Out1) -> Delay25/1
  Delay25/1 -> Adder Tree/1(In1)
  Product Array/2(Out2) -> Delay26/1
  Product Array/3(Out3) -> Delay27/1
  Product Array/4(Out4) -> Delay28/1
  Product Array/5(Out5) -> Delay29/1
  Product Array/6(Out6) -> Delay30/1
  Product Array/7(Out7) -> Delay31/1
  Product Array/9(Out9) -> Delay33/1
  Product Array/8(Out8) -> Delay32/1
  Product Array/10(validOut) -> Delay34/1
  Delay26/1 -> Adder Tree/2(In2)
  Delay27/1 -> Adder Tree/3(In3)
  Delay28/1 -> Adder Tree/4(In4)
  Delay29/1 -> Adder Tree/5(In5)
  Delay30/1 -> Adder Tree/6(In6)
  Delay31/1 -> Adder Tree/7(In7)
  Delay32/1 -> Adder Tree/8(In8)
  Delay33/1 -> Adder Tree/9(In9)
  Delay34/1 -> Adder Tree/10(validIn)
  Delay35/1 -> Data Type Conversion/1
  Delay36/1 -> ReLU/2(validIn)
  Delay37/1 -> MaxPooling/1(Stream_In)
  Delay38/1 -> MaxPooling/2(Stream_Valid)
  Delay41/1 -> OutData/1
  Delay39/1 -> OutValid/1
  Delay40/1 -> OutAdddess/1
